simulink library "AbsDiff"  (R2019b)
settings: Solver=VariableStepAuto  StartTime=0.0  StopTime=10.0  RelTol=1e-3
settings Model: Creator=hp  LastModifiedBy=hp

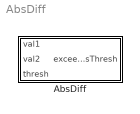
== system AbsDiff ==
  AbsDiff : Subsystem

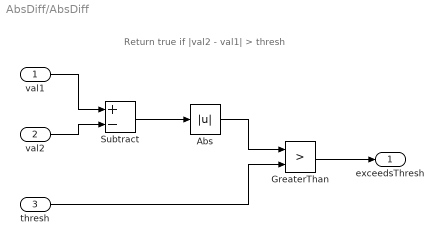
== system AbsDiff/AbsDiff ==
  note: Return true if |val2 - val1| > thresh
  val1 : Inport
  val2 : Inport  Port=2
  thresh : Inport  Port=3
  Abs : Abs
  GreaterThan : RelationalOperator  Operator=>  OutDataTypeStr=boolean  RndMeth=Simplest
  Subtract : Sum  Inputs=+-
  exceedsThresh : Outport
  wires:
  val1/1 -> Subtract/1
  Subtract/1 -> Abs/1
  Abs/1 -> GreaterThan/1
  val2/1 -> Subtract/2
  thresh/1 -> GreaterThan/2
  GreaterThan/1 -> exceedsThresh/1
